simulink model "lab3es1"  (R2021a)
settings: Solver=VariableStepAuto  StartTime=0.0  StopTime=10.0  RelTol=1e-3
settings Model: Creator=bonvoltnuovo  LastModifiedBy=bonvoltnuovo

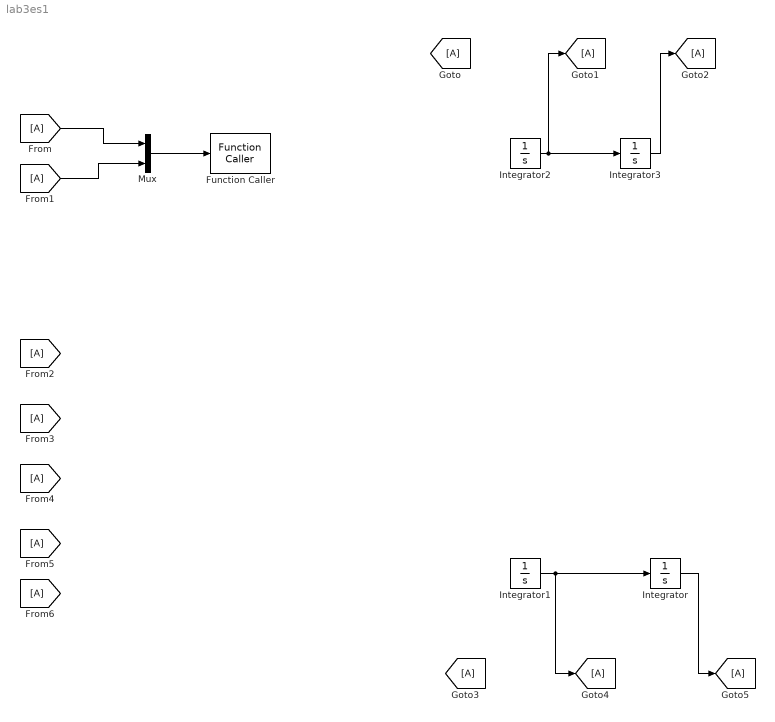
== system lab3es1 ==
  Function Caller : FunctionCaller  FunctionPrototype=y = f(u)  InputArgumentSpecifications=<Enter example>  OutputArgumentSpecifications=<Enter example>
  Integrator{,1..3} (4 alike) : Integrator
  Mux : Mux  Inputs=2
  wires:
  [A] -> Mux/2
  Mux/1 -> Function Caller/1
  [A] -> Mux/1
  Integrator2/1 -> Integrator3/1, [A]
  Integrator3/1 -> [A]
  Integrator/1 -> [A]
  Integrator1/1 -> Integrator/1, [A]
